simulink model "LVDAIN"  (R2021b)
settings: Solver=VariableStepAuto  StartTime=0.0  StopTime=10.0  RelTol=1e-3
settings Model: Creator=vince  LastModifiedBy=vince

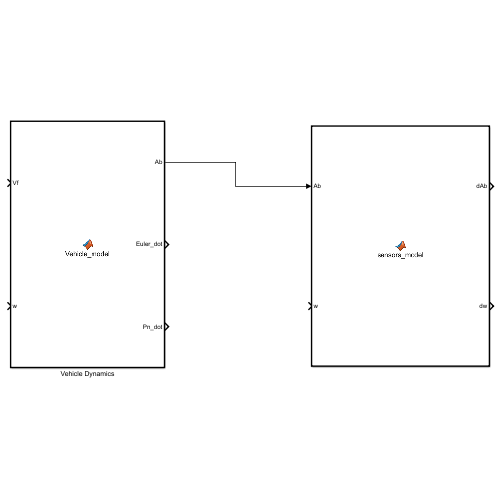
[thumbnail: Simulink's stored preview of the top-level diagram]
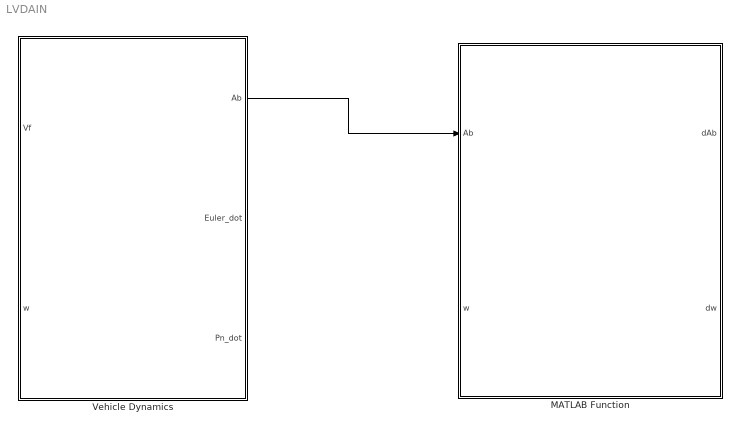
== system LVDAIN ==
  MATLAB Function : MATLAB Function  TreatAsAtomicUnit=on
  Vehicle Dynamics : MATLAB Function  TreatAsAtomicUnit=on
  wires:
  Vehicle Dynamics/1(Ab) -> MATLAB Function/1(Ab)

== matlab function LVDAIN/MATLAB Function ==
  data: Ab input; dAb output; w input; dw output
function [dAb, dw] = sensors_model(Ab, w)

%% Parameters

% Accelerometer
Ba = 0.02; % m/s^2
SFa = 0.05;
MISa = 0.1; % deg
stdv_a = 0.0055; % standard deviation
Wna = stdv_a*randn(3,1); % White Noise

Sa = [SFa MISa MISa;
      MISa SFa MISa;
      MISa MISa SFa];

% Gyros
Bg = 5; % deg/s
SFg = 0;
MISg = 0.1; % deg
stdv_g = 0.6325; % standard deviation
Wng = stdv_g*randn(3,1); % White Noise

Sg = [SFg MISg MISg;
      MISg SFg MISg;
      MISg MISg SFg];

%% Models

% Accelerometer
dAb = Ba*ones(3,1) + Sa * Ab + Wna;

% Gyros
dw = Bg*ones(3,1) + Sb * Ag + Wng;

== matlab function LVDAIN/Vehicle Dynamics ==
  data: Vf input; Ab output; w input; Euler_dot output; Pn_dot output
function [Ab, Euler_dot, Pn_dot] = Vehicle_model(Vf, w)
%% Land Vehicle Dynamic model
% x_dot is the derivative of x
wbx = w(1);
wby = w(2);
wbz = w(3);

% Model
Abx = Vf_dot + g*sin(theta);
Aby = Vf*wbz - g*sin(phi)*cos(theta);
Abz = -Vf*wby - g*cos(phi)*cos(theta);
phi_dot = wbx + sin(phi)*tan(theta)*wby + cos(phi)*tan(theta)*wbz;
theta_dot = cos(phi)*wby - sin(phi)*wbz;
psi_dot = sin(phi)/cos(theta)*wby + cos(phi)/cos(theta) * wbz;
Pnn_dot = Vf*cos(theta)*cos(psi);
Pne_dot = Vf*cos(theta)*sin(psi);
Pnd_dot = Vf*sin(theta);

Ab = [Abx, Aby, Abz]';
Euler_dot = [phi_dot, theta_dot, psi_dot]';
Pn_dot = [Pnn_dot, Pne_dot, Pnd_dot]';
